simulink model "MPC_with_disturbance__gungen_ibrahim"  (R2017a)
settings: Solver=ode45  StartTime=0.0  StopTime=3  RelTol=1e-3  EnableMultiTasking=on
libraries: mpclib x1, simulink x1
settings Model: Creator=igungen  LastModifiedBy=gunge
settings DataIOCC: LimitDataPoints=on  SaveFormat=Array
settings OptimizationCC: LifeSpan=inf
settings DebuggingCC: UnderspecifiedInitializationDetection=Classic  MergeDetectMultiDrivingBlocksExec=none  SolverPrmCheckMsg=warning  SFUnexpectedBacktrackingDiag=warning  SFNoUnconditionalDefaultTransitionDiag=warning  SFExecutionAtInitializationDiag=none
settings HardwareCC: ProdBitPerPointer=32  ProdBitPerSizeT=32  ProdBitPerPtrDiffT=32  ProdLargestAtomicFloat=None  ProdIntDivRoundTo=Undefined  ProdEndianess=Unspecified  ProdWordSize=32  ProdHWDeviceType=32-bit Generic
settings ModelReferenceCC: PropagateSignalLabelsOutOfModel=off
settings GRTTargetCC: TargetLangStandard=C89/C90 (ANSI)  GeneratePreprocessorConditionals=Disable all
settings ConfigComp: CovMetricSettings=dw  CovHtmlReporting=on  CovSaveCumulativeToWorkspaceVar=on  CovSaveSingleToWorkspaceVar=on  CovExternalEMLEnable=off

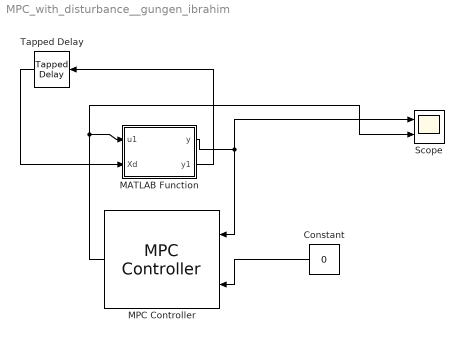
== system MPC_with_disturbance__gungen_ibrahim ==
  Constant : Constant  Value=0
  MATLAB Function : MATLAB Function  TreatAsAtomicUnit=on
  MPC Controller : mpclib/MPC Controller  mpcobj=mpc1  x0=[]  is_multiple=0  enable_value=0  return_u0=off  ref_from_ws=off  ref_signal_name=[]  ref_preview=off  md_from_ws=off  md_signal_name=[]  md_preview=off  from_project=off  project_file=MPCtask.mat  md_inport=off  mv_inport=off  cost_outport=off  return_sequence=off  return_qpstatus=off  return_state=off  state_inport=off  lims_inport=off  ywt_inport=off  is_designfromscratch=0  uwt_inport=off  duwt_inport=off  rhoeps_inport=off  uref_inport=off  n_ts=0.01  n_mv=1  n_md=0  n_ud=0  n_mo=1  n_uo=0  BlockDataType=double  SampleTimeInherited=off  switch_inport=off
  Scope : Scope  NumInputPorts=2
  Tapped Delay : simulink/Discrete/Tapped Delay  vinit=[0; 0; 0; 10]  samptime=-1  NumDelays=1  DelayOrder=Newest  includeCurrent=off
  wires:
  MATLAB Function/1(y) -> Scope/1, MPC Controller/1
  MPC Controller/1 -> Scope/2, MATLAB Function/1(u1)
  Constant/1 -> MPC Controller/2
  MATLAB Function/2(y1) -> Tapped Delay/1
  Tapped Delay/1 -> MATLAB Function/2(Xd)

== matlab function MPC_with_disturbance__gungen_ibrahim/MATLAB Function ==
  data: u1 input; Xd input; y output; y1 output
function [y,y1] = fcn(u1,Xd)
%#codegen
X1 = Xd;
A = [0.671440949146974 -0.0349851588312698 0 0;
    0.0517781225234599 0.734336221121412 0 0;
    0.00146077048938851 0.0430296983691291 1 0;
    1.25304060607981 0.434617178346022 1.50000000000000 1];

B = [0.138024770584345;2.47712399331690;0.0650504336464155;0.809483361601781];

C = [0 0 0 1];

D =[0];

p_diss = [0; 0; -30; 0];
R = 500; %m

X2 = A*X1+ B* u1 + p_diss*(1/R);
Y = C*X1 + D*u1;

y = Y;
y1 = X2;
